simulink model "pid_sl"  (R2014b)
settings: Solver=ode45  StartTime=0.0  StopTime=20  RelTol=1e-3
values from neighbouring files (symbols this model uses):
  b = 0.00007892    (= 7.892e-05)    [origin.m]    (also in reference.m)
  c = 0.063    [origin.m]    (also in reference.m = 0.63)
  g = 9.8    [origin.m]    (also in reference.m = 9.81)
  J = 0.0007176    [origin.m]
  l = 0.2    [origin.m]    (also in reference.m)
  m = 0.1    [origin.m]    (also in reference.m)
  M = 0.136    [origin.m]    (also in reference.m)
  PI = 3.14159265358979    (= 3.14159265359)    [origin.m]    (also in reference.m = 3.1415926536)
libraries: simulink x1
settings Model: Creator=Admin  LastModifiedBy=Admin

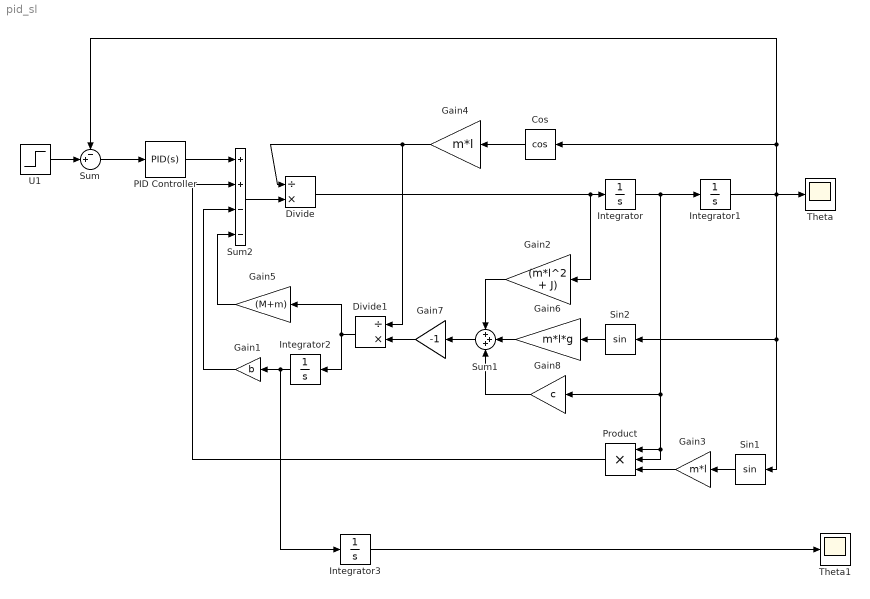
== system pid_sl ==
  " Cos" : Trigonometry  Operator=cos
  " Sin1" : Trigonometry
  " Sin2" : Trigonometry
  Divide : Product  Inputs=/*
  Divide1 : Product  Inputs=/*
  Gain1 : Gain  Gain=b
  Gain2 : Gain  Gain=(m*l^2 + J)
  Gain3 : Gain  Gain=m*l
  Gain4 : Gain  Gain=m*l
  Gain5 : Gain  Gain=(M+m)
  Gain6 : Gain  Gain=m*l*g
  Gain7 : Gain  Gain=-1
  Gain8 : Gain  Gain=c
  Integrator{,1..3} (4 alike) : Integrator
  PID Controller : simulink/Continuous/PID Controller  Controller=PID  TimeDomain=Continuous-time  SampleTime=-1  IntegratorMethod=Forward Euler  FilterMethod=Forward Euler  Form=Parallel  P=1  I=100  D=1  N=100  InitialConditionSource=internal  InitialConditionForIntegrator=0  InitialConditionForFilter=0  ExternalReset=none  LimitOutput=off  UpperSaturationLimit=inf  LowerSaturationLimit=-inf  LinearizeAsGain=on  AntiWindupMode=none  Kb=1  TrackingMode=off  Kt=1  PParamMin=[]  PParamMax=[]  IParamMin=[]  IParamMax=[]  DParamMin=[]  DParamMax=[]  NParamMin=[]  NParamMax=[]  KbParamMin=[]  KbParamMax=[]  KtParamMin=[]  KtParamMax=[]  POutMin=[]  POutMax=[]  IOutMin=[]  IOutMax=[]  DOutMin=[]  DOutMax=[]  NOutMin=[]  NOutMax=[]  KbOutMin=[]  KbOutMax=[]  KtOutMin=[]  KtOutMax=[]  IntegratorOutMin=[]  IntegratorOutMax=[]  FilterOutMin=[]  FilterOutMax=[]  SumOutMin=[]  SumOutMax=[]  SumI1OutMin=[]  SumI1OutMax=[]  SumI2OutMin=[]  SumI2OutMax=[]  SumI3OutMin=[]  SumI3OutMax=[]  SumDOutMin=[]  SumDOutMax=[]  SaturationOutMin=[]  SaturationOutMax=[]  IntegratorContinuousStateAttributes=''  IntegratorStateMustResolveToSignalObject=off  IntegratorRTWStateStorageClass=Auto  FilterContinuousStateAttributes=''  FilterStateMustResolveToSignalObject=off  FilterRTWStateStorageClass=Auto  DifferentiatorICPrevScaledInput=0  DifferentiatorOutMin=[]  DifferentiatorOutMax=[]  UseFilter=on
  Product : Product  Inputs=3
  Sum : Sum  Inputs=-+|
  Sum1 : Sum  Inputs=+++
  Sum2 : Sum  Inputs=++--
  Theta : Scope
      settings: TimeRange=10  YMin=-4  YMax=1
  Theta1 : Scope
      settings: TimeRange=20  YMin=0  YMax=2500
  U1 : Step  Time=0.1  After=PI  SampleTime=0
  wires:
  Integrator/1 -> Product/1, Product/2, Gain8/1, Integrator1/1
  Integrator2/1 -> Integrator3/1, Gain1/1
  Product/1 -> Sum2/2
  Integrator1/1 -> " Sin1"/1, " Sin2"/1, Theta/1, " Cos"/1, Sum/1
  Divide/1 -> Gain2/1, Integrator/1
  Sum2/1 -> Divide/2
  " Sin2"/1 -> Gain6/1
  Gain2/1 -> Sum1/1
  Gain6/1 -> Sum1/2
  Sum1/1 -> Gain7/1
  Divide1/1 -> Gain5/1, Integrator2/1
  Gain5/1 -> Sum2/4
  Gain1/1 -> Sum2/3
  Gain7/1 -> Divide1/2
  Integrator3/1 -> Theta1/1
  Gain8/1 -> Sum1/3
  Gain4/1 -> Divide1/1, Divide/1
  " Sin1"/1 -> Gain3/1
  " Cos"/1 -> Gain4/1
  Gain3/1 -> Product/3
  PID Controller/1 -> Sum2/1
  U1/1 -> Sum/2
  Sum/1 -> PID Controller/1
